simulink model "ExRobotAndEnvironmentControllerContPI"  (Simulink 8.9)
settings: Solver=ode45  StartTime=0.0  StopTime=1000  FixedStep=.01  RelTol=1e-3  EnableMultiTasking=on
values from neighbouring files (symbols this model uses):
  INITIAL_ROBOT_POS_THETA = 1.5*2    (= 3)    [InitRobotAndEnvironment.m]
  INITIAL_ROBOT_POS_X = 0    [InitRobotAndEnvironment.m]
  INITIAL_ROBOT_POS_Y = 0    [InitRobotAndEnvironment.m]
  INTER_WHEEL_DISTANCE = 0.12    [InitRobotAndEnvironment.m]
  ki_teta = omega*omega/alpha    (= 0.12)    [InitRobotAndEnvironment.m]
  kp_teta = 3*ksi*omega/alpha    (= 0.36)    [InitRobotAndEnvironment.m]
  MAX_SPEED = .5    (= 0.5)    [InitRobotAndEnvironment.m]
  Te = 0.05    [InitRobotAndEnvironment.m]
  ts = SENSOR_SAMPLING_TIME    (= 0.001)    [InitRobotAndEnvironment.m]
  ts_anim = ANIMATION_SAMPLING_TIME    (= 0.01)    [InitRobotAndEnvironment.m]
undefined symbols (not defined in the file or in its folder): Env, Robot, RobotInit
settings Model: SuppressorTable=22 serialization::archive 11 0 6 0 0 0 11 0  Creator=alex  LastModifiedBy=cathrind
settings DataIOCC: SignalLoggingSaveFormat=Dataset
settings OptimizationCC: ExpressionDepthLimit=2147483647
settings SFSimCC: SimParseCustomCode=off

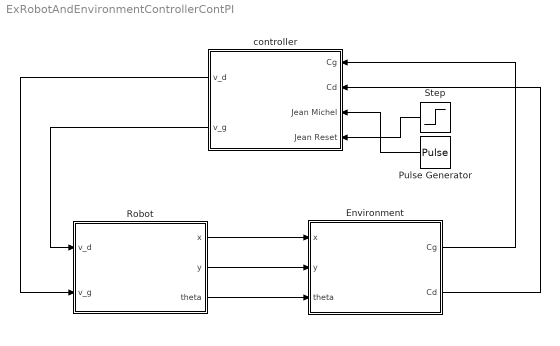
== system ExRobotAndEnvironmentControllerContPI ==
  Environment : Subsystem
  Pulse Generator : DiscretePulseGenerator  PulseType=Time based  Amplitude=1000  Period=3  PulseWidth=90
  Robot : Subsystem
  Step : Step  Before=1  After=0  SampleTime=Te
  controller : Subsystem
  wires:
  Robot/1(x) -> Environment/1(x)
  Robot/2(y) -> Environment/2(y)
  Robot/3(theta) -> Environment/3(theta)
  Environment/1(Cg) -> controller/1(Cg)
  Environment/2(Cd) -> controller/2(Cd)
  controller/1(v_d) -> Robot/2(v_g)
  controller/2(v_g) -> Robot/1(v_d)
  Pulse Generator/1 -> controller/3(Jean Michel)
  Step/1 -> controller/4(Jean Reset)

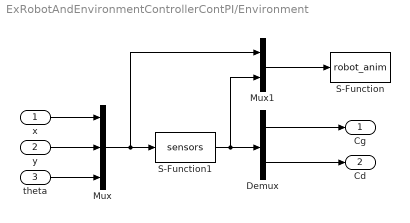
== system ExRobotAndEnvironmentControllerContPI/Environment ==
  x : Inport
  y : Inport  Port=2
  theta : Inport  Port=3
  Demux : Demux  Outputs=2
  Mux : Mux  Inputs=3
  Mux1 : Mux  Inputs=2
  S-Function : S-Function  FunctionName=robot_anim  Parameters=ts_anim,Env,Robot,RobotInit  SFunctionDeploymentMode=off  EnableBusSupport=off
  S-Function1 : S-Function  FunctionName=sensors  Parameters=ts,Env,Robot  SFunctionDeploymentMode=off  EnableBusSupport=off
  Cg : Outport
  Cd : Outport  Port=2
  wires:
  x/1 -> Mux/1
  y/1 -> Mux/2
  theta/1 -> Mux/3
  Mux/1 -> S-Function1/1, Mux1/1
  S-Function1/1 -> Mux1/2, Demux/1
  Mux1/1 -> S-Function/1
  Demux/1 -> Cg/1
  Demux/2 -> Cd/1

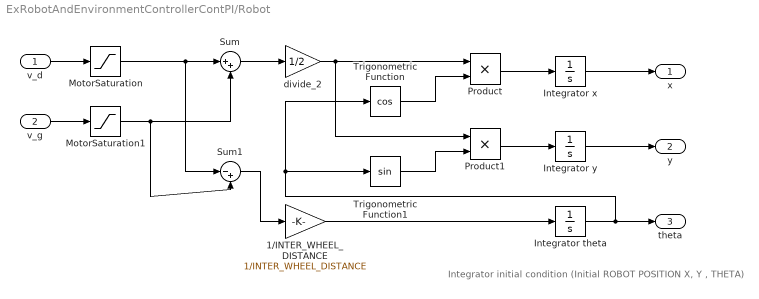
== system ExRobotAndEnvironmentControllerContPI/Robot ==
  note: Integrator initial condition (Initial ROBOT POSITION X, Y , THETA)
  v_d : Inport
  v_g : Inport  Port=2
  1/INTER_WHEEL_DISTANCE : Gain  Gain=1/INTER_WHEEL_DISTANCE
  Integrator theta : Integrator  InitialCondition=INITIAL_ROBOT_POS_THETA
  Integrator x : Integrator  InitialCondition=INITIAL_ROBOT_POS_X
  Integrator y : Integrator  InitialCondition=INITIAL_ROBOT_POS_Y
  MotorSaturation : Saturate  UpperLimit=MAX_SPEED  LowerLimit=-MAX_SPEED
  MotorSaturation1 : Saturate  UpperLimit=MAX_SPEED  LowerLimit=-MAX_SPEED
  Product : Product  RndMeth=Zero
  Product1 : Product  RndMeth=Zero
  Sum : Sum  Inputs=|++
  Sum1 : Sum  Inputs=|-+
  Trigonometric Function : Trigonometry  Operator=cos
  Trigonometric Function1 : Trigonometry
  divide_2 : Gain  Gain=1/2
  x : Outport
  y : Outport  Port=2
  theta : Outport  Port=3
  wires:
  v_d/1 -> MotorSaturation/1
  Integrator x/1 -> x/1
  Integrator y/1 -> y/1
  Integrator theta/1 -> Trigonometric Function/1, Trigonometric Function1/1, theta/1
  Sum/1 -> divide_2/1
  divide_2/1 -> Product1/1, Product/1
  Trigonometric Function/1 -> Product/2
  Trigonometric Function1/1 -> Product1/2
  Product/1 -> Integrator x/1
  Product1/1 -> Integrator y/1
  Sum1/1 -> 1/INTER_WHEEL_DISTANCE/1
  1/INTER_WHEEL_DISTANCE/1 -> Integrator theta/1
  v_g/1 -> MotorSaturation1/1
  MotorSaturation1/1 -> Sum/2, Sum1/2
  MotorSaturation/1 -> Sum/1, Sum1/1

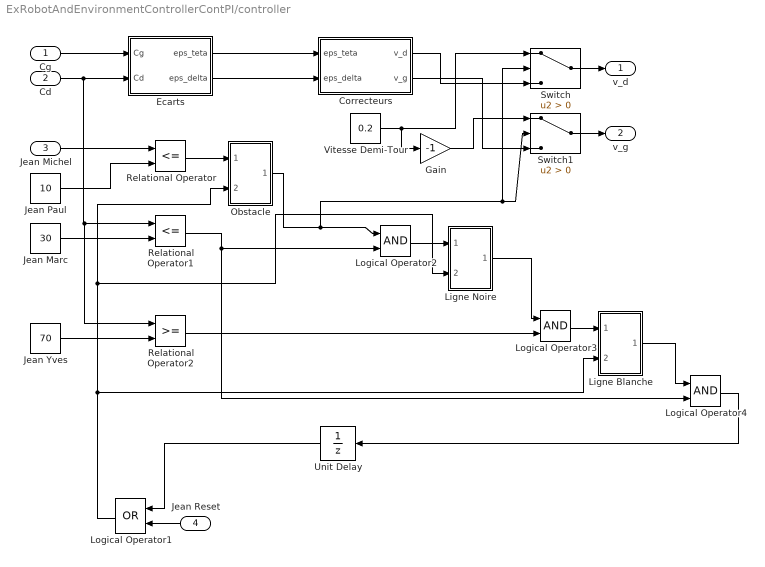
== system ExRobotAndEnvironmentControllerContPI/controller ==
  Cg : Inport
  Cd : Inport  Port=2
  Jean Michel : Inport  Port=3
  Jean Reset : Inport  Port=4
  Correcteurs : Subsystem
  Ecarts : Subsystem
  Gain : Gain  Gain=-1
  Jean Marc : Constant  Value=30  OutDataTypeStr=single
  Jean Paul : Constant  Value=10  OutDataTypeStr=uint32
  Jean Yves : Constant  Value=70  OutDataTypeStr=single
  Ligne Blanche : Subsystem
  Ligne Noire : Subsystem
  Logical Operator1 : Logic  Operator=OR  AllPortsSameDT=off  OutDataTypeStr=boolean
  Logical Operator2 : Logic  AllPortsSameDT=off  OutDataTypeStr=boolean
  Logical Operator3 : Logic  AllPortsSameDT=off  OutDataTypeStr=boolean
  Logical Operator4 : Logic  AllPortsSameDT=off  OutDataTypeStr=boolean
  Obstacle : Subsystem
  Relational Operator : RelationalOperator  Operator=<=  OutDataTypeStr=boolean  RndMeth=Simplest
  Relational Operator1 : RelationalOperator  Operator=<=  OutDataTypeStr=boolean  RndMeth=Simplest
  Relational Operator2 : RelationalOperator  OutDataTypeStr=boolean  RndMeth=Simplest
  Switch : Switch  Criteria=u2 > Threshold
  Switch1 : Switch  Criteria=u2 > Threshold
  Unit Delay : UnitDelay  SampleTime=-1
  Vitesse Demi-Tour : Constant  Value=0.2  OutDataTypeStr=single
  v_d : Outport
  v_g : Outport  Port=2
  wires:
  Ecarts/2(eps_delta) -> Correcteurs/2(eps_delta)
  Cg/1 -> Ecarts/1(Cg)
  Cd/1 -> Relational Operator2/1, Relational Operator1/1, Ecarts/2(Cd)
  Ecarts/1(eps_teta) -> Correcteurs/1(eps_teta)
  Switch/1 -> v_d/1
  Switch1/1 -> v_g/1
  Vitesse Demi-Tour/1 -> Switch/1, Gain/1
  Jean Michel/1 -> Relational Operator/1
  Jean Paul/1 -> Relational Operator/2
  Jean Marc/1 -> Relational Operator1/2
  Relational Operator1/1 -> Logical Operator2/2, Logical Operator4/2
  Correcteurs/1(v_d) -> Switch/3
  Gain/1 -> Switch1/1
  Correcteurs/2(v_g) -> Switch1/3
  Relational Operator/1 -> Obstacle/1(Set)
  Obstacle/1(Out) -> Switch/2, Switch1/2, Logical Operator2/1
  Logical Operator2/1 -> Ligne Noire/1(Set)
  Relational Operator2/1 -> Logical Operator3/2
  Ligne Noire/1(Out) -> Logical Operator3/1
  Logical Operator3/1 -> Ligne Blanche/1(Set)
  Ligne Blanche/1(Out) -> Logical Operator4/1
  Jean Yves/1 -> Relational Operator2/2
  Logical Operator4/1 -> Unit Delay/1
  Unit Delay/1 -> Logical Operator1/1
  Logical Operator1/1 -> Ligne Blanche/2(Reset), Ligne Noire/2(Reset), Obstacle/2(Reset)
  Jean Reset/1 -> Logical Operator1/2

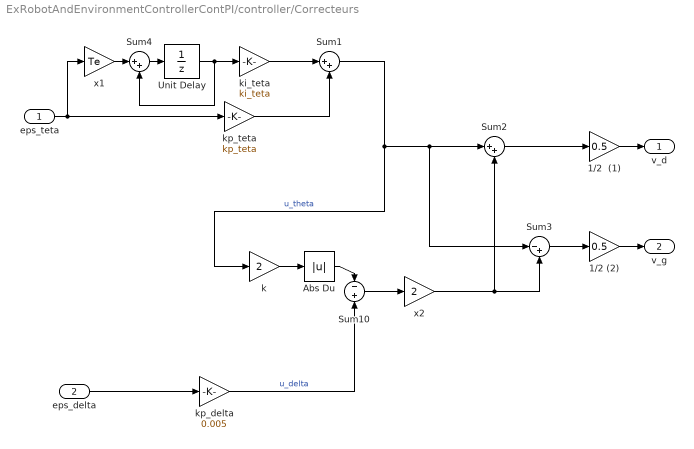
== system ExRobotAndEnvironmentControllerContPI/controller/Correcteurs ==
  eps_teta : Inport
  eps_delta : Inport  Port=2
  1/2  (1) : Gain  Gain=0.5  SaturateOnIntegerOverflow=on  OutDataTypeStr=Inherit: Same as input  ParamDataTypeStr=Inherit: Same as input
  1/2 (2) : Gain  Gain=0.5  SaturateOnIntegerOverflow=on  OutDataTypeStr=Inherit: Same as input  ParamDataTypeStr=Inherit: Same as input
  Abs Du : Abs  SaturateOnIntegerOverflow=on
  Sum1 : Sum  Inputs=|++  SaturateOnIntegerOverflow=on
  Sum10 : Sum  Inputs=-+  SaturateOnIntegerOverflow=on
  Sum2 : Sum  Inputs=|++  SaturateOnIntegerOverflow=on
  Sum3 : Sum  Inputs=|-+  SaturateOnIntegerOverflow=on
  Sum4 : Sum  Inputs=|++  SaturateOnIntegerOverflow=on
  Unit Delay : UnitDelay  SampleTime=-1
  k : Gain  Gain=2  SaturateOnIntegerOverflow=on  OutDataTypeStr=Inherit: Same as input  ParamDataTypeStr=Inherit: Same as input
  ki_teta : Gain  Gain=ki_teta  SaturateOnIntegerOverflow=on  OutDataTypeStr=Inherit: Same as input  ParamDataTypeStr=Inherit: Same as input
  kp_delta : Gain  Gain=0.005
  kp_teta : Gain  Gain=kp_teta  SaturateOnIntegerOverflow=on  OutDataTypeStr=Inherit: Same as input  ParamDataTypeStr=Inherit: Same as input
  x1 : Gain  Gain=Te  SaturateOnIntegerOverflow=on  OutDataTypeStr=Inherit: Same as input  ParamDataTypeStr=Inherit: Same as input
  x2 : Gain  Gain=2  SaturateOnIntegerOverflow=on  OutDataTypeStr=Inherit: Same as input  ParamDataTypeStr=Inherit: Same as input
  v_d : Outport
  v_g : Outport  Port=2
  wires:
  ki_teta/1 -> Sum1/1
  kp_teta/1 -> Sum1/2
  Sum2/1 -> 1/2  (1)/1
  Sum3/1 -> 1/2 (2)/1
  k/1 -> Abs Du/1
  kp_delta/1 -> Sum10/2  "u_delta"
  Abs Du/1 -> Sum10/1
  x2/1 -> Sum2/2, Sum3/2
  Sum10/1 -> x2/1
  Sum1/1 -> k/1, Sum2/1, Sum3/1  "u_theta"
  1/2  (1)/1 -> v_d/1
  1/2 (2)/1 -> v_g/1
  eps_delta/1 -> kp_delta/1
  eps_teta/1 -> x1/1, kp_teta/1
  Sum4/1 -> Unit Delay/1
  x1/1 -> Sum4/1
  Unit Delay/1 -> Sum4/2, ki_teta/1

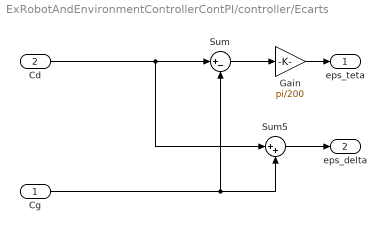
== system ExRobotAndEnvironmentControllerContPI/controller/Ecarts ==
  Cg : Inport
  Cd : Inport  Port=2
  Gain : Gain  Gain=pi/200
  Sum : Sum  Inputs=|+-
  Sum5 : Sum  Inputs=|++
  eps_teta : Outport
  eps_delta : Outport  Port=2
  wires:
  Sum/1 -> Gain/1
  Cd/1 -> Sum/1, Sum5/1
  Cg/1 -> Sum/2, Sum5/2
  Gain/1 -> eps_teta/1
  Sum5/1 -> eps_delta/1

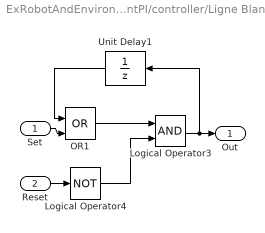
== system ExRobotAndEnvironmentControllerContPI/controller/Ligne Blanche ==
  Set : Inport
  Reset : Inport  Port=2
  Logical Operator3 : Logic  AllPortsSameDT=off  OutDataTypeStr=boolean
  Logical Operator4 : Logic  Operator=NOT  AllPortsSameDT=off  OutDataTypeStr=boolean
  OR1 : Logic  Operator=OR  IconShape=distinctive  AllPortsSameDT=off  OutDataTypeStr=boolean
  Unit Delay1 : UnitDelay  SampleTime=-1
  Out : Outport
  wires:
  Unit Delay1/1 -> OR1/1
  Logical Operator4/1 -> Logical Operator3/2
  Reset/1 -> Logical Operator4/1
  Set/1 -> OR1/2
  OR1/1 -> Logical Operator3/1
  Logical Operator3/1 -> Out/1, Unit Delay1/1

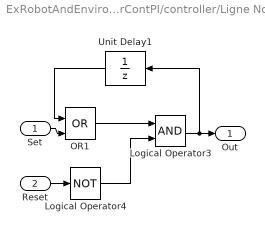
== system ExRobotAndEnvironmentControllerContPI/controller/Ligne Noire ==
  Set : Inport
  Reset : Inport  Port=2
  Logical Operator3 : Logic  AllPortsSameDT=off  OutDataTypeStr=boolean
  Logical Operator4 : Logic  Operator=NOT  AllPortsSameDT=off  OutDataTypeStr=boolean
  OR1 : Logic  Operator=OR  IconShape=distinctive  AllPortsSameDT=off  OutDataTypeStr=boolean
  Unit Delay1 : UnitDelay  SampleTime=-1
  Out : Outport
  wires:
  Unit Delay1/1 -> OR1/1
  Logical Operator4/1 -> Logical Operator3/2
  Reset/1 -> Logical Operator4/1
  Set/1 -> OR1/2
  OR1/1 -> Logical Operator3/1
  Logical Operator3/1 -> Out/1, Unit Delay1/1

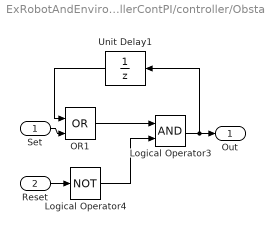
== system ExRobotAndEnvironmentControllerContPI/controller/Obstacle ==
  Set : Inport
  Reset : Inport  Port=2
  Logical Operator3 : Logic  AllPortsSameDT=off  OutDataTypeStr=boolean
  Logical Operator4 : Logic  Operator=NOT  AllPortsSameDT=off  OutDataTypeStr=boolean
  OR1 : Logic  Operator=OR  IconShape=distinctive  AllPortsSameDT=off  OutDataTypeStr=boolean
  Unit Delay1 : UnitDelay  SampleTime=-1
  Out : Outport
  wires:
  Unit Delay1/1 -> OR1/1
  Logical Operator4/1 -> Logical Operator3/2
  Reset/1 -> Logical Operator4/1
  Set/1 -> OR1/2
  OR1/1 -> Logical Operator3/1
  Logical Operator3/1 -> Out/1, Unit Delay1/1
